simulink model "PippoSchema"  (R2024a)
settings: Solver=VariableStepAuto  StartTime=0.0  StopTime=13.1  RelTol=1e-3
settings Model: Creator=Stefano  LastModifiedBy=stefanopanzieri
settings SolverCC: AlgebraicLoopSolver=TrustRegion
settings DebuggingCC: UnconnectedInputMsg=warning  UnconnectedOutputMsg=warning  UnconnectedLineMsg=warning
settings ModelReferenceCC: EnableRefExpFcnMdlSchedulingChecks=on
settings SFSimCC: CustomCodeUndefinedFunction=UseInterfaceOnly
settings RTWCC: GPUComputeCapability=3.5  DLArmComputeVersion=19.05

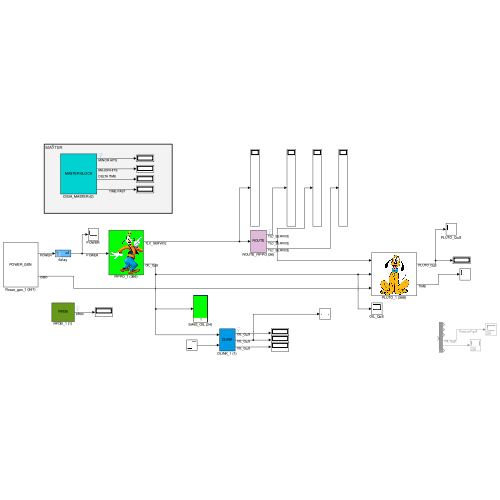
[thumbnail: Simulink's stored preview of the top-level diagram]
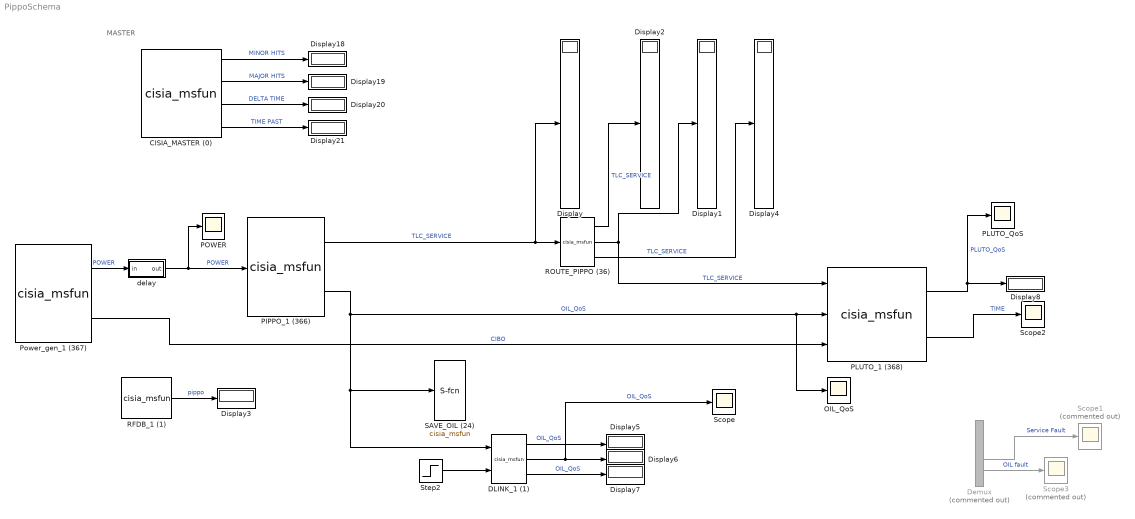
== system PippoSchema ==
  note: MASTER
  CISIA_MASTER (0) : M-S-Function  FunctionName=cisia_msfun  Parameters=Parameter1, Parameter2, Parameter3, resources, Parameter4, Parameter5, Parameter6, Parameter7, Parameter8, Parameter9,Parameter11,Parameter12  mask(S-function:msfcn_unit_delay){Parameter1='CISIA_MASTER', Parameter2=[1 6 12], Parameter3='Pippo', resources=on, Parameter4=on, Parameter5=off, Parameter6=off, Parameter7=off, Parameter8=0.001, Parameter9=off, Parameter11=on, Parameter12=on}
      mask prompts: Parameter1 "entity name"; Parameter2 "sampling time"; Parameter3 "project"; resources "Save status at each major hit"; Parameter4 "Show Operative Levels with colors"; Parameter5 "Load Entities from file"; Parameter6 "Load Start from Mask"; Parameter7 "Real Time"; Parameter8 "Real Time Hit (sec)"; Parameter9 "Skip saving"; Parameter11 "Show unconnected"; Parameter12 "Save port values"
      mask help:
      | MASTER BLOCK
      | v.2.0
      mask Display: disp('MASTER BLOCK')
  DLINK_1 (1) : M-S-Function  FunctionName=cisia_msfun  Parameters=Parameter1, Parameter2, Parameter3, Parameter4, Parameter5, Parameter6, Parameter7  mask(S-function:msfcn_unit_delay){Parameter1='DLINK_1', Parameter2=1, Parameter3='SistemiIoT', Parameter4=3, Parameter5=0, Parameter6=1, Parameter7=on}
      mask prompts: Parameter1 "entity name"; Parameter2 "sampling time"; Parameter3 "project"; Parameter4 "number of output links"; Parameter5 "default value for outputs"; Parameter6 "link dimension"; Parameter7 "select link from input"
      mask help: This is a level-2 MATLAB file S-function which demonstrates CISIA entity
      mask Display: disp('DLINK')
  Demux : Demux  Commented=on  Outputs=6
  Display{,1..8,18..21} (13 alike) : Display
  OIL_QoS : Scope
  PIPPO_1 (366) : M-S-Function  FunctionName=cisia_msfun  Parameters=Parameter1, Parameter2, Parameter3, resources, Parameter10, codeupdate, step_received, step_computed, dynamic_computed, step_sended, id_entity, id_project, id_type, name_type, color  mask(S-function:msfcn_unit_delay){Parameter1='PIPPO_1', Parameter2=1, Parameter3='', resources=, Parameter10=off, codeupdate=off, step_received=|, step_computed=, dynamic_computed=, step_sended=|, id_entity=366, id_project=28, id_type=100, name_type=PIPPO, color=#FFFFFF}
      mask step_received=|
      | Operative_Level=min([POWER 1-Mechanical_Fault 1-max(Cyber_Fault)]);
      |
      | TLC_services=TLC_services_init;
      mask step_sended=|
      | OIL_QoS=Operative_Level;
      |
      |
      | TLC_SERVICE=TLC_services;
      mask prompts: Parameter1 "entity name"; Parameter2 "sampling time"; Parameter3 "project"; resources "input resources and state variables"; Parameter10 "Bring state variables to output"; codeupdate "update code from mask"
      mask help: This is a level-2 MATLAB file S-function which demonstrates CISIA entity
      mask DialogControl Container1 Prompt: All parameters
      mask Display: image('Icons/PIPPO.png')
  PLUTO_1 (368) : M-S-Function  FunctionName=cisia_msfun  Parameters=Parameter1, Parameter2, Parameter3, resources, Parameter10, codeupdate, step_received, step_computed, dynamic_computed, step_sended, id_entity, id_project, id_type, name_type, color  mask(S-function:msfcn_unit_delay){Parameter1='PLUTO_1', Parameter2=1, Parameter3='', resources=, Parameter10=off, codeupdate=off, step_received=|, step_computed=, dynamic_computed=, step_sended=|, id_entity=368, id_project=28, id_type=102, name_type=PLUTO, color=#FFFFFF}
      mask step_received=|
      | Service_Fault=max(abs(Consumed_Services.*TLC_SERVICE-Consumed_Services));
      |
      | OIL_buffer=push_buffer(OIL_QoS,OIL_buffer);
      |
      |
      | Oil_Fault=1-delayed(OIL_buffer,3,1);
      |
      |
      | Operative_Level=min([1-Oil_Fault 1-Service_Fault]);
      mask step_sended=|
      | PLUTO_QoS=Operative_Level;
      |
      | TIME=block.CurrentTime;
      mask prompts: Parameter1 "entity name"; Parameter2 "sampling time"; Parameter3 "project"; resources "input resources and state variables"; Parameter10 "Bring state variables to output"; codeupdate "update code from mask"
      mask help: This is a level-2 MATLAB file S-function which demonstrates CISIA entity
      mask DialogControl Container1 Prompt: All parameters
      mask Display: image('Icons/PLUTO.png')
  PLUTO_QoS : Scope
  POWER : Scope
  Power_gen_1 (367) : M-S-Function  FunctionName=cisia_msfun  Parameters=Parameter1, Parameter2, Parameter3, resources, Parameter10, codeupdate, step_received, step_computed, dynamic_computed, step_sended, id_entity, id_project, id_type, name_type, color  mask(S-function:msfcn_unit_delay){Parameter1='Power_gen_1', Parameter2=1, Parameter3='', resources=, Parameter10=off, codeupdate=off, step_received=, step_computed=, dynamic_computed=, step_sended=POWER=min([Operative_Level 1-Mechanical_Fault]);, id_entity=367, id_project=28, id_type=101, name_type=POWER_GEN, color=#FFFFFF}
      mask prompts: Parameter1 "entity name"; Parameter2 "sampling time"; Parameter3 "project"; resources "input resources and state variables"; Parameter10 "Bring state variables to output"; codeupdate "update code from mask"
      mask help: This is a level-2 MATLAB file S-function which demonstrates CISIA entity
      mask DialogControl Container1 Prompt: All parameters
      mask Display: disp('POWER_GEN')
  RFDB_1 (1) : M-S-Function  FunctionName=cisia_msfun  Parameters=Parameter1, Parameter2, Parameter3, Parameter4, Parameter5  mask(S-function:msfcn_unit_delay){Parameter1='RFDB_1', Parameter2=1, Parameter3='SistemiIoT', Parameter4='pippo', Parameter5='REAL'}
      mask prompts: Parameter1 "entity name"; Parameter2 "sampling time"; Parameter3 "project"; Parameter4 "variable name"; Parameter5 "variable type"
      mask help: This is a level-2 MATLAB file S-function which demonstrates CISIA entity
      mask Display: disp('RFDB')
  ROUTE_PIPPO (36) : M-S-Function  FunctionName=cisia_msfun  Parameters=Parameter1, Parameter2, Parameter3, Parameter4, Parameter5, Parameter6, Parameter7  mask(S-function:msfcn_unit_delay){Parameter1='ROUTE_PIPPO', Parameter2=1, Parameter3='ORO', Parameter4=3, Parameter5=0, Parameter6=20, Parameter7=off}
      mask prompts: Parameter1 "entity name"; Parameter2 "sampling time"; Parameter3 "project"; Parameter4 "number of output links"; Parameter5 "default value for outputs"; Parameter6 "link dimension (unused))"; Parameter7 "select resource elements and output port from input"
      mask help: This is a level-2 MATLAB file S-function which demonstrates CISIA entity
      mask Display: disp('ROUTE')
  SAVE_OIL (24) : M-S-Function  FunctionName=cisia_msfun  Parameters=Parameter1, Parameter2, Parameter3, Parameter4,Parameter5,Parameter6,Parameter7  mask(S-function:msfcn_unit_delay){Parameter1='SAVE_OIL', Parameter2=1, Parameter3='Iside', Parameter4=on, Parameter5=[1], Parameter6=[1], Parameter7=off}
      mask prompts: Parameter1 "entity name"; Parameter2 "sampling time"; Parameter3 "project"; Parameter4 "display bars"; Parameter5 "values"; Parameter6 "logic"; Parameter7 "display B/W"
      mask help: This is a level-2 MATLAB file S-function which demonstrates CISIA entity
      mask DialogControl Container3 Prompt: Display
      mask Display:
      | display=get_param(gcb, 'Parameter4');
      | greymap=get_param(gcb, 'Parameter7');
      | 
      | if strcmp(display,'on')
      | 
      |     val=str2num(get_param(gcb, 'Parameter5'));
      |     logic=str2num(get_param(gcb, 'Parameter6'));
      |     n=length(val);
      | 
      |     val2=val;
      |     l=length(logic);
      |     if l>0
      |         for i=1:l
      |             if logic(i)==-1
      |                 val2(i)=1-val2(i);
      |             end
      |         end
      |     end
      | 
      | 
      | 
      | 
      |     if strcmp(greymap,'on')
      |         val_r=round(val2*50)+1;
      |         colormap=gray(60);
      |         color2=[0 0 0];
      |     else
      |         val_r=round(val2*20)+1;
      |         colormap=hsv(60);
      |         color2=[0 0 1];
      |     end
      | 
      |     patch([0 0 n n], [0 -0.2 -0.2 0], [1 1 1]);
      | 
      |     for i=1:n
      |         color=colormap(val_r(i),:);
      |         patch([i-1 i-1 i i],[0 1 1 0],color)
      |         patch([i-1 i],[val(i) val(i)],color2)
      | 
      |     end
      | 
      |     for i=1:n
      |         patch([i i], [-0.2 1], [0 0 0]);
      |         text(i-0.5, -0.1, num2str(val(i)));
      |     end
      | 
      | 
      | else
      | 
      |     disp('SAVE');
      | 
      | end
  Scope : Scope
  Scope1 : Scope  Commented=on
  Scope2 : Scope
  Scope3 : Scope  Commented=on
  Step2 : Step  Before=1  After=2  SampleTime=1
  delay : Subsystem  mask{delay=0.9, output=ones(1,1)}
  wires:
  CISIA_MASTER (0)/1 -> Display18/1  "MINOR HITS"
  CISIA_MASTER (0)/2 -> Display19/1  "MAJOR HITS"
  CISIA_MASTER (0)/4 -> Display21/1  "TIME PAST"
  CISIA_MASTER (0)/3 -> Display20/1  "DELTA TIME"
  Power_gen_1 (367)/1 -> delay/1(in)  "POWER"
  PIPPO_1 (366)/2 -> SAVE_OIL (24)/1, DLINK_1 (1)/1, OIL_QoS/1, PLUTO_1 (368)/2  "OIL_QoS"
  PIPPO_1 (366)/1 -> ROUTE_PIPPO (36)/1, Display/1  "TLC_SERVICE"
  ROUTE_PIPPO (36)/2 -> PLUTO_1 (368)/1, Display1/1  "TLC_SERVICE"
  ROUTE_PIPPO (36)/1 -> Display2/1  "TLC_SERVICE"
  DLINK_1 (1)/1 -> Display5/1  "OIL_QoS"
  DLINK_1 (1)/2 -> Scope/1, Display6/1  "OIL_QoS"
  Step2/1 -> DLINK_1 (1)/2
  DLINK_1 (1)/3 -> Display7/1  "OIL_QoS"
  RFDB_1 (1)/1 -> Display3/1  "pippo"
  ROUTE_PIPPO (36)/3 -> Display4/1  "TLC_SERVICE"
  PLUTO_1 (368)/1 -> PLUTO_QoS/1, Display8/1  "PLUTO_QoS"
  PLUTO_1 (368)/2 -> Scope2/1  "TIME"
  Demux/5 -> Scope3/1  "OIL fault"
  delay/1(out) -> POWER/1, PIPPO_1 (366)/1  "POWER"
  Demux/4 -> Scope1/1  "Service Fault"
  Power_gen_1 (367)/2 -> PLUTO_1 (368)/3  "CIBO"

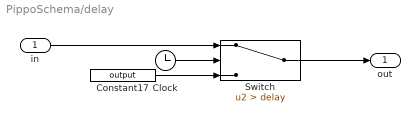
== system PippoSchema/delay ==
  in : Inport
  Clock : Clock
  Constant17 : Constant  Value=output
  Switch : Switch  Criteria=u2 > Threshold  Threshold=delay  SaturateOnIntegerOverflow=off  InputSameDT=off
  out : Outport
  wires:
  Switch/1 -> out/1
  Constant17/1 -> Switch/3
  in/1 -> Switch/1
  Clock/1 -> Switch/2
